simulink library "csu_mkf_multiplicative_update_mtv_lib"  (R2014b)
settings: Solver=ode45  SolverMode=SingleTasking  StartTime=0.0  StopTime=10.0  RelTol=1e-3
values from neighbouring files (symbols this model uses):
  kfl_central_body_rotation_rate = central_body_rotation_rate    [csc_kfl_kalman_filter_mtv_init.m]
undefined symbols (not defined in the file or in its folder): fcv_acquiring, fcv_diverged, fcv_initializing, mkf_cov_jam_index, mkf_cov_jam_matrix, mkf_null_quat, mkf_zero_gibbs
libraries: util_quat_lib x5, util_common_lib x4, simulink x2, util_info_lib x1, util_fsw_frame_rotation_lib x1
settings Model: ExtModeAutoUpdateStatusClock=off  Creator=escrane  LastModifiedBy=tgorton

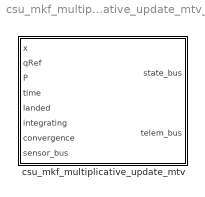
== system csu_mkf_multiplicative_update_mtv_lib ==
  csu_mkf_multiplicative_update_mtv : Subsystem

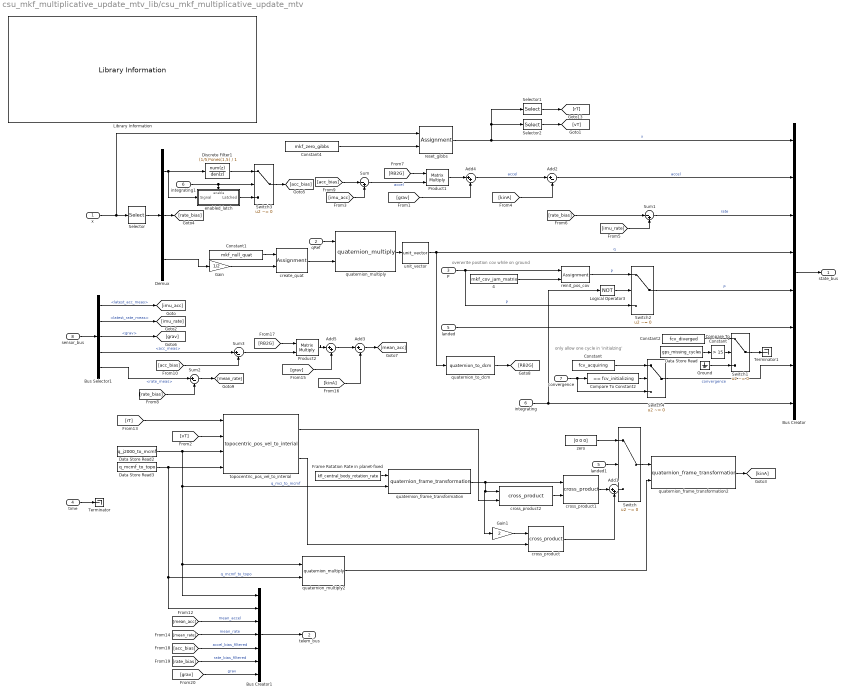
== system csu_mkf_multiplicative_update_mtv_lib/csu_mkf_multiplicative_update_mtv ==
  note: only allow one cycle in 'initialzing'
  note: overwrite position cov while on ground
  x : Inport
  qRef : Inport  Port=2
  P : Inport  Port=3
  time : Inport  Port=4
  landed : Inport  Port=5
  integrating : Inport  Port=6
  convergence : Inport  Port=7
  sensor_bus : Inport  Port=8
  "      4" : Constant  Value=mkf_cov_jam_matrix
  Add1 : Sum  Inputs=|++
  Add2 : Sum  Inputs=|+-
  Add3 : Sum  Inputs=|+-
  Add4 : Sum  Inputs=|++
  Add5 : Sum  Inputs=|++
  Bus Creator : BusCreator  Inputs=8
  Bus Creator1 : BusCreator  Inputs=7
  Bus Selector1 : BusSelector  OutputSignals=latest_acc_meas,latest_rate_meas,grav,acc_meas,rate_meas
  Compare To Constant : simulink/Logic and Bit Operations/Compare To Constant  relop=>  const=15  OutDataTypeStr=boolean
  Compare To Constant2 : simulink/Logic and Bit Operations/Compare To Constant  relop===  const=fcv_initializing  OutDataTypeStr=boolean
  Constant : Constant  Value=fcv_acquiring  OutDataTypeStr=double
  Constant1 : Constant  Value=mkf_null_quat
  Constant2 : Constant  Value=fcv_diverged  OutDataTypeStr=double
  Constant4 : Constant  Value=mkf_zero_gibbs
  Data Store Read : DataStoreRead  DataStoreName=gps_missing_cycles
  Data Store Read2 : DataStoreRead  DataStoreName=q_j2000_to_mcmf
  Data Store Read3 : DataStoreRead  DataStoreName=q_mcmf_to_topo
  Demux : Demux  Outputs=[3 3 3]
  Discrete Filter1 : DiscreteFilter  Numerator=(1/5)*ones(1,5)  Denominator=1
  Frame Rotation Rate in planet-fixed : Constant  Value=kfl_central_body_rotation_rate
  Gain : Gain  Gain=1/2
  Gain1 : Gain  Gain=2
  Ground : Ground
  Library Information : util_info_lib/Library Information  owner='NONE'
  Logical Operator3 : Logic  Operator=NOT  AllPortsSameDT=off  OutDataTypeStr=boolean
  Product1 : Product  Multiplication=Matrix(*)  RndMeth=Zero
  Product2 : Product  Multiplication=Matrix(*)  RndMeth=Zero
  Selector : Selector  InputPortWidth=kfl_n_state  Indices=mkf_selection_index
  Selector1 : Selector  InputPortWidth=kfl_n_state  Indices=kfl_pos_index
  Selector2 : Selector  InputPortWidth=kfl_n_state  Indices=kfl_vel_index
  Sum : Sum  Inputs=|-+
  Sum1 : Sum  Inputs=|-+
  Sum2 : Sum  Inputs=|+-
  Sum3 : Sum  Inputs=|+-
  Switch : Switch  Criteria=u2 ~= 0
  Switch1 : Switch  Criteria=u2 ~= 0  Threshold=0.5  InputSameDT=on
  Switch2 : Switch  Criteria=u2 ~= 0
  Switch3 : Switch  Criteria=u2 ~= 0
  Switch4 : Switch  Criteria=u2 ~= 0  Threshold=0.5  InputSameDT=on
  Terminator : Terminator
  Terminator1 : Terminator
  create_quat : Assignment  Indices=[1 2 3]
  cross_product : util_common_lib/cross_product  SystemSampleTime=-1
  cross_product1 : util_common_lib/cross_product  SystemSampleTime=-1
  cross_product2 : util_common_lib/cross_product  SystemSampleTime=-1
  enabled_latch : Subsystem
  integrating1 : InportShadow  Port=6
  landed1 : InportShadow  Port=5
  quaternion_frame_transformation : util_quat_lib/quaternion_frame_transformation  SystemSampleTime=-1
  quaternion_frame_transformation2 : util_quat_lib/quaternion_frame_transformation  SystemSampleTime=-1
  quaternion_multiply : util_quat_lib/quaternion_multiply  SystemSampleTime=-1
  quaternion_multiply2 : util_quat_lib/quaternion_multiply  SystemSampleTime=-1
  quaternion_to_dcm : util_quat_lib/quaternion_to_dcm  SystemSampleTime=-1
  reinit_pos_cov : Assignment  NumberOfDimensions=2  IndexOptions=Index vector (dialog),Index vector (dialog)  Indices=mkf_cov_jam_index,mkf_cov_jam_index  OutputSizes=1,1
  reset_gibbs : Assignment  Indices=kfl_gibbs_index
  topocentric_pos_vel_to_interial : util_fsw_frame_rotation_lib/topocentric_pos_vel_to_interial  SystemSampleTime=-1
  unit_vector : util_common_lib/unit_vector  SystemSampleTime=-1
  zero : Constant  Value=[0 0 0]
  state_bus : Outport
  telem_bus : Outport  Port=2
  wires:
  [grav] -> Bus Creator1/7  "grav"
  Switch1/1 -> Terminator1/1
  Ground/1 -> Switch1/3
  Constant2/1 -> Switch1/1
  Discrete Filter1/1 -> Switch3/1
  enabled_latch/1(Latched) -> Switch3/3
  integrating1/1 -> enabled_latch/Enable, Switch3/2
  Switch3/1 -> [acc_bias]
  Demux/1 -> enabled_latch/1(Signal), Discrete Filter1/1
  cross_product/1 -> Add1/2
  topocentric_pos_vel_to_interial/2 -> cross_product/2
  Data Store Read2/1 -> topocentric_pos_vel_to_interial/3, quaternion_multiply2/1, Bus Creator1/1, quaternion_frame_transformation/2  "q_mci_to_mcmf"
  [rT] -> topocentric_pos_vel_to_interial/1
  [vT] -> topocentric_pos_vel_to_interial/2
  [kinA] -> Add2/2
  Add2/1 -> Bus Creator/2  "accel"
  Add4/1 -> Add2/1  "accel"
  cross_product1/1 -> Add1/1
  cross_product2/1 -> cross_product1/2
  Gain1/1 -> cross_product/1
  quaternion_frame_transformation/1 -> cross_product1/1, Gain1/1, cross_product2/1
  Selector2/1 -> [vT]
  Selector1/1 -> [rT]
  Data Store Read3/1 -> topocentric_pos_vel_to_interial/4, Bus Creator1/2, quaternion_multiply2/2  "q_mcmf_to_topo"
  Frame Rotation Rate in planet-fixed/1 -> quaternion_frame_transformation/1
  [grav] -> Add4/2
  [RB2G] -> Product1/1
  quaternion_to_dcm/1 -> [RB2G]
  Sum/1 -> Product1/2  "accel"
  unit_vector/1 -> Bus Creator/4, quaternion_to_dcm/1  "q"
  Gain/1 -> create_quat/2
  Constant1/1 -> create_quat/1
  quaternion_multiply/1 -> unit_vector/1
  Constant4/1 -> reset_gibbs/2
  Sum1/1 -> Bus Creator/3  "rate"
  reset_gibbs/1 -> Selector1/1, Selector2/1, Bus Creator/1  "x"
  [imu_rate] -> Sum1/2
  [imu_acc] -> Sum/2
  Bus Selector1/1 -> [imu_acc]  "<latest_acc_meas>"
  sensor_bus/1 -> Bus Selector1/1
  Selector/1 -> Demux/1
  time/1 -> Terminator/1
  Bus Creator/1 -> state_bus/1
  Demux/3 -> Gain/1
  qRef/1 -> quaternion_multiply/1
  create_quat/1 -> quaternion_multiply/2
  Demux/2 -> [rate_bias]
  P/1 -> Switch2/3, reinit_pos_cov/1  "P"
  landed/1 -> Bus Creator/6
  reinit_pos_cov/1 -> Switch2/1  "P"
  Switch2/1 -> Bus Creator/5  "P"
  "      4"/1 -> reinit_pos_cov/2
  topocentric_pos_vel_to_interial/1 -> cross_product2/2
  Switch/1 -> quaternion_frame_transformation2/1
  quaternion_frame_transformation2/1 -> [kinA]
  quaternion_multiply2/1 -> quaternion_frame_transformation2/2
  convergence/1 -> Switch4/3, Compare To Constant2/1
  Compare To Constant2/1 -> Switch4/2
  Constant/1 -> Switch4/1
  Bus Selector1/3 -> [grav]  "<grav>"
  Bus Selector1/4 -> Sum3/1  "<acc_meas>"
  Bus Selector1/5 -> Sum2/1  "<rate_meas>"
  Bus Selector1/2 -> [imu_rate]  "<latest_rate_meas>"
  [rate_bias] -> Sum1/1
  Sum2/1 -> [mean_rate]
  [rate_bias] -> Sum2/2
  [acc_bias] -> Sum/1
  [acc_bias] -> Sum3/2
  Sum3/1 -> Product2/2
  [mean_rate] -> Bus Creator1/4  "mean_rate"
  [mean_acc] -> Bus Creator1/3  "mean_accel"
  Bus Creator1/1 -> telem_bus/1
  [kinA] -> Add3/2
  Add5/1 -> Add3/1
  Product2/1 -> Add5/1
  [RB2G] -> Product2/1
  Add3/1 -> [mean_acc]
  [grav] -> Add5/2
  zero/1 -> Switch/1
  landed1/1 -> Switch/2
  Add1/1 -> Switch/3
  Product1/1 -> Add4/1
  integrating/1 -> Logical Operator3/1, Bus Creator/8
  Logical Operator3/1 -> Switch2/2
  [acc_bias] -> Bus Creator1/5  "accel_bias_filtered"
  [rate_bias] -> Bus Creator1/6  "rate_bias_filtered"
  x/1 -> reset_gibbs/1, Selector/1
  Data Store Read/1 -> Compare To Constant/1
  Compare To Constant/1 -> Switch1/2
  Switch4/1 -> Bus Creator/7  "convergence"

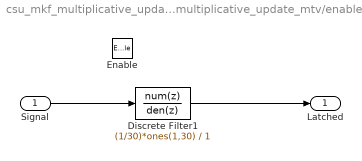
== system csu_mkf_multiplicative_update_mtv_lib/csu_mkf_multiplicative_update_mtv/enabled_latch ==
  Signal : Inport
  Enable : EnablePort
  Discrete Filter1 : DiscreteFilter  Numerator=(1/30)*ones(1,30)  Denominator=1
  Latched : Outport
  wires:
  Discrete Filter1/1 -> Latched/1
  Signal/1 -> Discrete Filter1/1
